simulink model "CMPE243finalprojectdesign0x2DYi0x011Fit_Avar"  (R2023b)
settings: Solver=VariableStepAuto  StartTime=0.0  StopTime=10000  RelTol=1e-3
libraries: simulink_extras x6, embmathops x2, hdlsllib x1
settings Model: PacingRate=5  Creator=berkenulusoy  LastModifiedBy=ASUS TUF

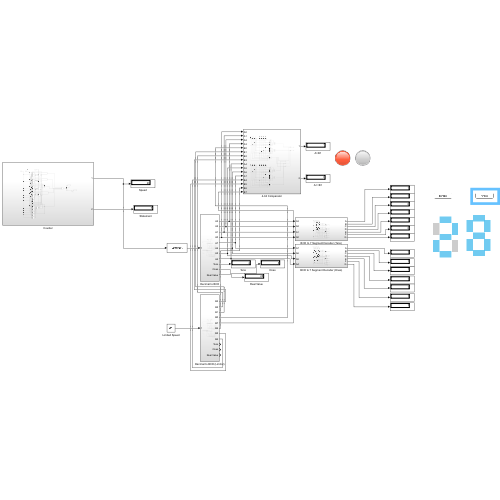
[thumbnail: Simulink's stored preview of the top-level diagram]
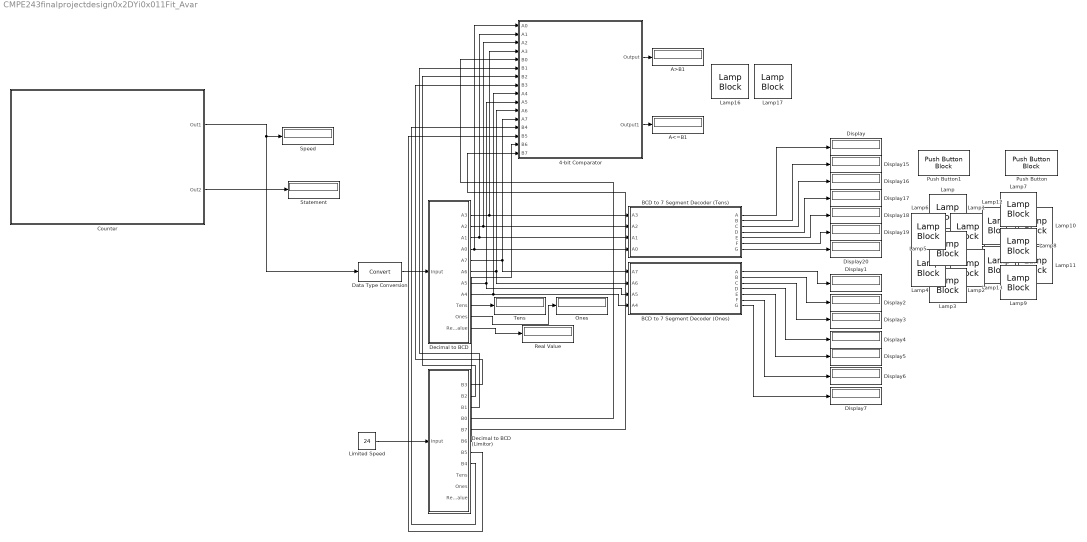
== system CMPE243finalprojectdesign0x2DYi0x011Fit_Avar ==
  4-bit Comparator : Subsystem
  A<=B1 : Display
  A>B1 : Display
  BCD to 7 Segment Decoder (Ones) : Subsystem
  BCD to 7 Segment Decoder (Tens) : Subsystem
  Counter : Subsystem
  Data Type Conversion : DataTypeConversion  SaturateOnIntegerOverflow=off  RndMeth=Floor
  Decimal to BCD : Subsystem
  Decimal to BCD (Limitor) : Subsystem
  Display{,1..7,15..20} (14 alike) : Display
  Lamp{,1..13} (14 alike) : LampBlock  LabelPosition=Hide  Icon=Rectangle
  Lamp16 : LampBlock  LabelPosition=Hide
  Lamp17 : LampBlock  LabelPosition=Hide
  Limited Speed : Constant  Value=24
  Ones : Display
  Push Button : PushButtonBlock  ButtonText=increase  OffValue=0.000000
  Push Button1 : PushButtonBlock  ButtonText=decrease  OffValue=0.000000
  Real Value : Display
  Speed : Display
  Statement : Display
  Tens : Display
  wires:
  Decimal to BCD/9(Tens) -> Tens/1
  Decimal to BCD/10(Ones) -> Ones/1
  Decimal to BCD/11(Real Value) -> Real Value/1
  BCD to 7 Segment Decoder (Ones)/6(F) -> Display6/1
  BCD to 7 Segment Decoder (Tens)/2(B) -> Display15/1
  BCD to 7 Segment Decoder (Ones)/2(B) -> Display2/1
  BCD to 7 Segment Decoder (Ones)/1(A) -> Display1/1
  BCD to 7 Segment Decoder (Tens)/7(G) -> Display20/1
  BCD to 7 Segment Decoder (Ones)/5(E) -> Display5/1
  BCD to 7 Segment Decoder (Ones)/4(D) -> Display4/1
  BCD to 7 Segment Decoder (Ones)/7(G) -> Display7/1
  BCD to 7 Segment Decoder (Tens)/1(A) -> Display/1
  BCD to 7 Segment Decoder (Tens)/5(E) -> Display18/1
  BCD to 7 Segment Decoder (Tens)/3(C) -> Display16/1
  BCD to 7 Segment Decoder (Tens)/4(D) -> Display17/1
  BCD to 7 Segment Decoder (Tens)/6(F) -> Display19/1
  BCD to 7 Segment Decoder (Ones)/3(C) -> Display3/1
  Decimal to BCD/1(A3) -> 4-bit Comparator/4(A3), BCD to 7 Segment Decoder (Tens)/1(A3)
  Decimal to BCD/2(A2) -> 4-bit Comparator/3(A2), BCD to 7 Segment Decoder (Tens)/2(A2)
  Decimal to BCD/4(A0) -> 4-bit Comparator/1(A0), BCD to 7 Segment Decoder (Tens)/4(A0)
  Decimal to BCD/5(A7) -> 4-bit Comparator/12(A7), BCD to 7 Segment Decoder (Ones)/1(A7)
  Decimal to BCD/6(A6) -> 4-bit Comparator/11(A6), BCD to 7 Segment Decoder (Ones)/2(A6)
  Decimal to BCD/7(A5) -> 4-bit Comparator/10(A5), BCD to 7 Segment Decoder (Ones)/3(A5)
  Decimal to BCD/8(A4) -> 4-bit Comparator/9(A4), BCD to 7 Segment Decoder (Ones)/4(A4)
  4-bit Comparator/2(Output1) -> A<=B1/1
  4-bit Comparator/1(Output) -> A>B1/1
  Decimal to BCD/3(A1) -> 4-bit Comparator/2(A1), BCD to 7 Segment Decoder (Tens)/3(A1)
  Data Type Conversion/1 -> Decimal to BCD/1(Input)
  Counter/2(Out2) -> Statement/1
  Counter/1(Out1) -> Data Type Conversion/1, Speed/1
  Decimal to BCD (Limitor)/1(B3) -> 4-bit Comparator/8(B3)
  Decimal to BCD (Limitor)/2(B2) -> 4-bit Comparator/7(B2)
  Decimal to BCD (Limitor)/3(B1) -> 4-bit Comparator/6(B1)
  Decimal to BCD (Limitor)/4(B0) -> 4-bit Comparator/5(B0)
  Decimal to BCD (Limitor)/5(B7) -> 4-bit Comparator/16(B7)
  Decimal to BCD (Limitor)/6(B6) -> 4-bit Comparator/15(B6)
  Decimal to BCD (Limitor)/7(B5) -> 4-bit Comparator/14(B5)
  Decimal to BCD (Limitor)/8(B4) -> 4-bit Comparator/13(B4)
  Limited Speed/1 -> Decimal to BCD (Limitor)/1(Input)

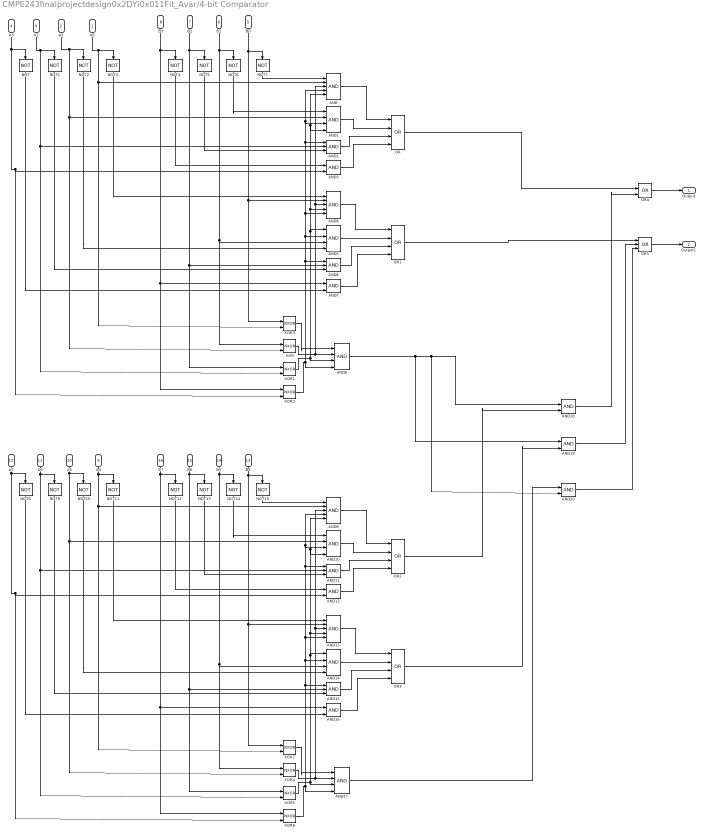
== system CMPE243finalprojectdesign0x2DYi0x011Fit_Avar/4-bit Comparator ==
  A0 : Inport
  A1 : Inport  Port=2
  A2 : Inport  Port=3
  A3 : Inport  Port=4
  B0 : Inport  Port=5
  B1 : Inport  Port=6
  B2 : Inport  Port=7
  B3 : Inport  Port=8
  A4 : Inport  Port=9
  A5 : Inport  Port=10
  A6 : Inport  Port=11
  A7 : Inport  Port=12
  B4 : Inport  Port=13
  B5 : Inport  Port=14
  B6 : Inport  Port=15
  B7 : Inport  Port=16
  AND{,4,9,13} (4 alike) : Logic  Inputs=5  IconShape=distinctive  AllPortsSameDT=off  OutDataTypeStr=boolean
  AND{1,5,8,10,14,17} (6 alike) : Logic  Inputs=4  IconShape=distinctive  AllPortsSameDT=off  OutDataTypeStr=boolean
  AND{2,6,11,15} (4 alike) : Logic  Inputs=3  IconShape=distinctive  AllPortsSameDT=off  OutDataTypeStr=boolean
  AND{3,7,12,16,18..20} (7 alike) : Logic  IconShape=distinctive  AllPortsSameDT=off  OutDataTypeStr=boolean
  NOT{,1..15} (16 alike) : Logic  Operator=NOT  IconShape=distinctive  AllPortsSameDT=off  OutDataTypeStr=boolean
  OR{,1..3} (4 alike) : Logic  Operator=OR  Inputs=4  IconShape=distinctive  AllPortsSameDT=off  OutDataTypeStr=boolean
  OR4 : Logic  Operator=OR  IconShape=distinctive  AllPortsSameDT=off  OutDataTypeStr=boolean
  OR5 : Logic  Operator=OR  Inputs=3  IconShape=distinctive  AllPortsSameDT=off  OutDataTypeStr=boolean
  XOR{,1..7} (8 alike) : Logic  Operator=NXOR  IconShape=distinctive  AllPortsSameDT=off  OutDataTypeStr=boolean
  Output : Outport
  Output1 : Outport  Port=2
  wires:
  NOT12/1 -> AND12/1
  AND12/1 -> OR2/4
  NOT14/1 -> AND10/1
  AND9/1 -> OR2/1
  XOR3/1 -> AND8/1
  OR1/1 -> OR5/1
  AND17/1 -> AND20/1
  AND16/1 -> OR3/4
  AND1/1 -> OR/2
  NOT1/1 -> AND6/3
  NOT11/1 -> AND13/1
  XOR7/1 -> AND17/1
  B1/1 -> NOT6/1, XOR/1, AND5/3
  AND2/1 -> OR/3
  B4/1 -> NOT15/1, XOR7/1, AND13/2
  B7/1 -> NOT12/1, XOR6/1, AND16/1
  NOT4/1 -> AND3/1
  AND4/1 -> OR1/1
  OR/1 -> OR4/1
  NOT9/1 -> AND15/3
  NOT5/1 -> AND2/3
  AND14/1 -> OR3/2
  OR3/1 -> AND19/2
  XOR/1 -> AND8/2, AND4/3, AND/3
  NOT7/1 -> AND/1
  A6/1 -> NOT9/1, XOR5/2, AND11/2
  NOT3/1 -> AND4/1
  A7/1 -> NOT8/1, XOR6/2, AND12/2
  OR5/1 -> Output1/1
  NOT8/1 -> AND16/2
  A2/1 -> NOT1/1, XOR1/2, AND2/2
  AND5/1 -> OR1/2
  XOR5/1 -> AND14/1, AND13/4, AND10/4, AND9/5, AND17/3
  NOT13/1 -> AND11/3
  AND6/1 -> OR1/3
  AND3/1 -> OR/4
  B3/1 -> NOT4/1, XOR2/1, AND7/1
  AND15/1 -> OR3/3
  B2/1 -> NOT5/1, XOR1/1, AND6/2
  AND8/1 -> AND19/1, AND20/2, AND18/1
  NOT/1 -> AND7/2
  AND10/1 -> OR2/2
  A4/1 -> NOT11/1, XOR7/2, AND9/2
  NOT15/1 -> AND9/1
  AND7/1 -> OR1/4
  A5/1 -> NOT10/1, XOR4/2, AND10/2
  XOR6/1 -> AND17/4, AND15/1, AND14/2, AND13/5, AND11/1, AND10/3, AND9/4
  B0/1 -> NOT7/1, XOR3/1, AND4/2
  NOT6/1 -> AND1/1
  AND/1 -> OR/1
  A0/1 -> NOT3/1, XOR3/2, AND/2
  A3/1 -> NOT/1, XOR2/2, AND3/2
  NOT10/1 -> AND14/4
  OR2/1 -> AND18/2
  AND19/1 -> OR5/2
  B5/1 -> NOT14/1, XOR4/1, AND14/3
  B6/1 -> NOT13/1, XOR5/1, AND15/2
  AND13/1 -> OR3/1
  XOR4/1 -> AND17/2, AND13/3, AND9/3
  XOR1/1 -> AND5/1, AND4/4, AND1/4, AND/5, AND8/3
  XOR2/1 -> AND8/4, AND6/1, AND5/2, AND4/5, AND2/1, AND1/3, AND/4
  OR4/1 -> Output/1
  AND11/1 -> OR2/3
  A1/1 -> NOT2/1, XOR/2, AND1/2
  AND18/1 -> OR4/2
  NOT2/1 -> AND5/4
  AND20/1 -> OR5/3

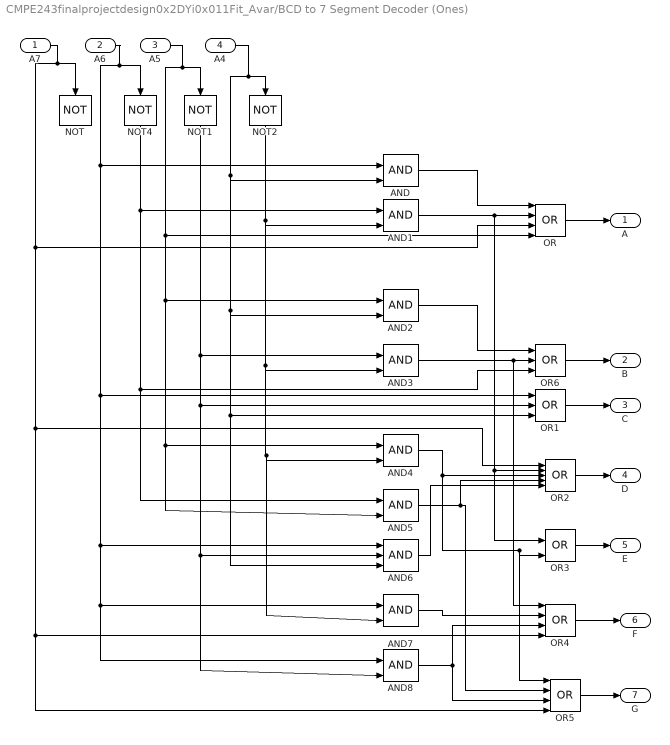
== system CMPE243finalprojectdesign0x2DYi0x011Fit_Avar/BCD to 7 Segment Decoder (Ones) ==
  A7 : Inport
  A6 : Inport  Port=2
  A5 : Inport  Port=3
  A4 : Inport  Port=4
  AND{,1..5,7..8} (8 alike) : Logic  IconShape=distinctive  AllPortsSameDT=off  OutDataTypeStr=boolean
  AND6 : Logic  Inputs=3  IconShape=distinctive  AllPortsSameDT=off  OutDataTypeStr=boolean
  NOT{,1..2,4} (4 alike) : Logic  Operator=NOT  IconShape=distinctive  AllPortsSameDT=off  OutDataTypeStr=boolean
  OR : Logic  Operator=OR  Inputs=4  IconShape=distinctive  AllPortsSameDT=off  OutDataTypeStr=boolean
  OR1 : Logic  Operator=OR  Inputs=3  IconShape=distinctive  AllPortsSameDT=off  OutDataTypeStr=boolean
  OR2 : Logic  Operator=OR  Inputs=5  IconShape=distinctive  AllPortsSameDT=off  OutDataTypeStr=boolean
  OR3 : Logic  Operator=OR  IconShape=distinctive  AllPortsSameDT=off  OutDataTypeStr=boolean
  OR4 : Logic  Operator=OR  Inputs=4  IconShape=distinctive  AllPortsSameDT=off  OutDataTypeStr=boolean
  OR5 : Logic  Operator=OR  Inputs=4  IconShape=distinctive  AllPortsSameDT=off  OutDataTypeStr=boolean
  OR6 : Logic  Operator=OR  Inputs=3  IconShape=distinctive  AllPortsSameDT=off  OutDataTypeStr=boolean
  A : Outport
  B : Outport  Port=2
  C : Outport  Port=3
  D : Outport  Port=4
  E : Outport  Port=5
  F : Outport  Port=6
  G : Outport  Port=7
  wires:
  OR5/1 -> G/1
  A7/1 -> NOT/1, OR/3, OR4/4, OR5/4, OR2/1
  AND8/1 -> OR4/3, OR5/3
  AND3/1 -> OR4/1, OR6/2
  NOT4/1 -> AND1/1, OR6/3, AND5/1
  AND1/1 -> OR2/2, OR3/1, OR/2
  AND5/1 -> OR2/4, OR5/2
  AND/1 -> OR/1
  AND7/1 -> OR4/2
  OR4/1 -> F/1
  OR6/1 -> B/1
  OR3/1 -> E/1
  NOT2/1 -> AND1/2, AND3/2, AND7/2, AND4/2
  AND2/1 -> OR6/1
  AND6/1 -> OR2/5
  A5/1 -> NOT1/1, OR/4, AND2/1, AND4/1, AND5/2
  OR2/1 -> D/1
  NOT1/1 -> AND3/1, OR1/2, AND6/2, AND8/2
  OR1/1 -> C/1
  A4/1 -> NOT2/1, AND/2, AND2/2, OR1/3, AND6/3
  A6/1 -> NOT4/1, AND/1, OR1/1, AND6/1, AND7/1, AND8/1
  AND4/1 -> OR2/3, OR5/1, OR3/2
  OR/1 -> A/1

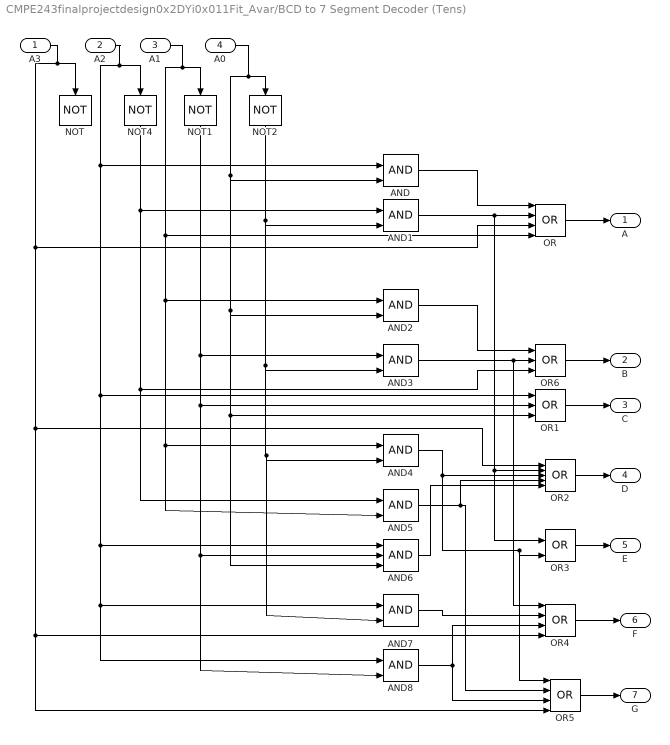
== system CMPE243finalprojectdesign0x2DYi0x011Fit_Avar/BCD to 7 Segment Decoder (Tens) ==
  A3 : Inport
  A2 : Inport  Port=2
  A1 : Inport  Port=3
  A0 : Inport  Port=4
  AND{,1..5,7..8} (8 alike) : Logic  IconShape=distinctive  AllPortsSameDT=off  OutDataTypeStr=boolean
  AND6 : Logic  Inputs=3  IconShape=distinctive  AllPortsSameDT=off  OutDataTypeStr=boolean
  NOT{,1..2,4} (4 alike) : Logic  Operator=NOT  IconShape=distinctive  AllPortsSameDT=off  OutDataTypeStr=boolean
  OR : Logic  Operator=OR  Inputs=4  IconShape=distinctive  AllPortsSameDT=off  OutDataTypeStr=boolean
  OR1 : Logic  Operator=OR  Inputs=3  IconShape=distinctive  AllPortsSameDT=off  OutDataTypeStr=boolean
  OR2 : Logic  Operator=OR  Inputs=5  IconShape=distinctive  AllPortsSameDT=off  OutDataTypeStr=boolean
  OR3 : Logic  Operator=OR  IconShape=distinctive  AllPortsSameDT=off  OutDataTypeStr=boolean
  OR4 : Logic  Operator=OR  Inputs=4  IconShape=distinctive  AllPortsSameDT=off  OutDataTypeStr=boolean
  OR5 : Logic  Operator=OR  Inputs=4  IconShape=distinctive  AllPortsSameDT=off  OutDataTypeStr=boolean
  OR6 : Logic  Operator=OR  Inputs=3  IconShape=distinctive  AllPortsSameDT=off  OutDataTypeStr=boolean
  A : Outport
  B : Outport  Port=2
  C : Outport  Port=3
  D : Outport  Port=4
  E : Outport  Port=5
  F : Outport  Port=6
  G : Outport  Port=7
  wires:
  OR5/1 -> G/1
  A3/1 -> NOT/1, OR/3, OR4/4, OR5/4, OR2/1
  AND8/1 -> OR4/3, OR5/3
  AND3/1 -> OR4/1, OR6/2
  NOT4/1 -> AND1/1, OR6/3, AND5/1
  AND1/1 -> OR2/2, OR3/1, OR/2
  AND5/1 -> OR2/4, OR5/2
  AND/1 -> OR/1
  AND7/1 -> OR4/2
  OR4/1 -> F/1
  OR6/1 -> B/1
  OR3/1 -> E/1
  NOT2/1 -> AND1/2, AND3/2, AND7/2, AND4/2
  AND2/1 -> OR6/1
  AND6/1 -> OR2/5
  A1/1 -> NOT1/1, OR/4, AND2/1, AND4/1, AND5/2
  OR2/1 -> D/1
  NOT1/1 -> AND3/1, OR1/2, AND6/2, AND8/2
  OR1/1 -> C/1
  A0/1 -> NOT2/1, AND/2, AND2/2, OR1/3, AND6/3
  A2/1 -> NOT4/1, AND/1, OR1/1, AND6/1, AND7/1, AND8/1
  AND4/1 -> OR2/3, OR5/1, OR3/2
  OR/1 -> A/1

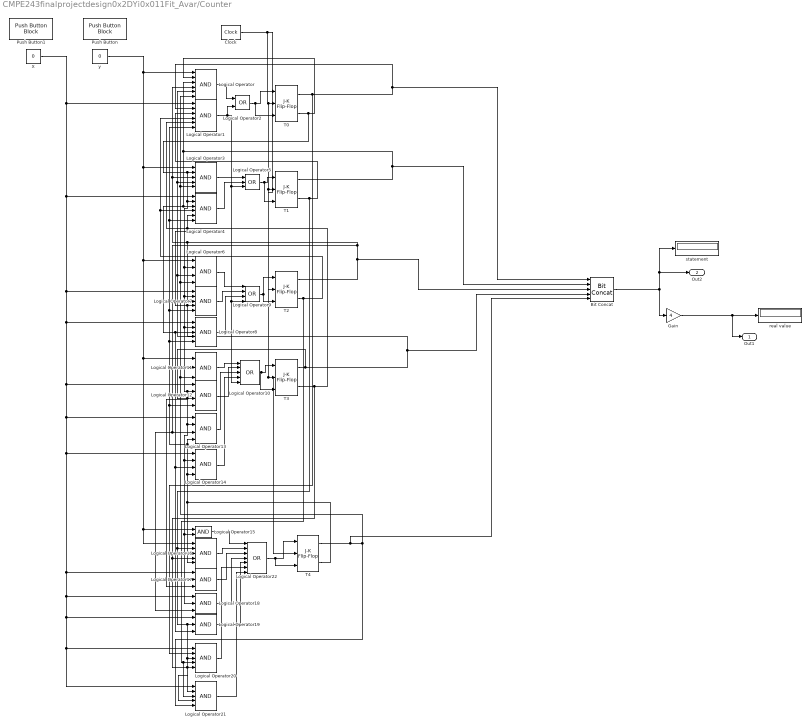
== system CMPE243finalprojectdesign0x2DYi0x011Fit_Avar/Counter ==
  Bit Concat : hdlsllib/Logic and Bit Operations/Bit Concat  numInputs=5
  Clock : simulink_extras/Flip Flops/Clock  period=1
  Gain : Gain  Gain=4
  Logical Operator : Logic  Inputs=6  AllPortsSameDT=off  OutDataTypeStr=boolean
  Logical Operator1 : Logic  Inputs=6  AllPortsSameDT=off  OutDataTypeStr=boolean
  Logical Operator10 : Logic  Operator=OR  Inputs=5  AllPortsSameDT=off  OutDataTypeStr=boolean
  Logical Operator{11,17..19} (4 alike) : Logic  Inputs=3  AllPortsSameDT=off  OutDataTypeStr=boolean
  Logical Operator{6,12..14} (4 alike) : Logic  Inputs=4  AllPortsSameDT=off  OutDataTypeStr=boolean
  Logical Operator15 : Logic  AllPortsSameDT=off  OutDataTypeStr=boolean
  Logical Operator{3,7..8,16,20..21} (6 alike) : Logic  Inputs=5  AllPortsSameDT=off  OutDataTypeStr=boolean
  Logical Operator2 : Logic  Operator=OR  AllPortsSameDT=off  OutDataTypeStr=boolean
  Logical Operator22 : Logic  Operator=OR  Inputs=7  AllPortsSameDT=off  OutDataTypeStr=boolean
  Logical Operator4 : Logic  Inputs=6  AllPortsSameDT=off  OutDataTypeStr=boolean
  Logical Operator5 : Logic  Operator=OR  Inputs=3  AllPortsSameDT=off  OutDataTypeStr=boolean
  Logical Operator9 : Logic  Operator=OR  Inputs=4  AllPortsSameDT=off  OutDataTypeStr=boolean
  Push Button : PushButtonBlock  ButtonText=increase  OffValue=0.000000
  Push Button1 : PushButtonBlock  ButtonText=decrease  OffValue=0.000000
  T{0..4} (5 alike) : simulink_extras/Flip Flops/J-K Flip-Flop  initial_condition=0
  X : Constant  Value=0
  real value : Display
  statement : Display
  y : Constant  Value=0
  Out1 : Outport
  Out2 : Outport  Port=2
  wires:
  X/1 -> Logical Operator1/1, Logical Operator4/1, Logical Operator7/1, Logical Operator8/1, Logical Operator12/1, Logical Operator13/1, Logical Operator14/1, Logical Operator17/1, Logical Operator19/1, Logical Operator21/1, Logical Operator20/1, Logical Operator18/1
  y/1 -> Logical Operator/1, Logical Operator3/1, Logical Operator6/1, Logical Operator11/1, Logical Operator15/1, Logical Operator16/1
  Logical Operator/1 -> Logical Operator2/1
  Logical Operator2/1 -> T0/3, T0/1
  T0/2 -> Logical Operator4/2, Logical Operator18/2, Logical Operator17/2, Logical Operator15/2, Logical Operator14/2, Logical Operator13/2, Logical Operator12/2, Logical Operator11/2, Logical Operator8/2, Logical Operator7/2, Logical Operator6/2, Logical Operator3/2, Logical Operator/2
  T1/2 -> Logical Operator16/2, Logical Operator21/2, Logical Operator20/3, Logical Operator19/2, Logical Operator1/3
  T2/2 -> Logical Operator16/3, Logical Operator20/4, Logical Operator21/3, Logical Operator4/4, Logical Operator1/4
  T3/2 -> Logical Operator16/4, Logical Operator21/4, Logical Operator20/5, Logical Operator8/4, Logical Operator7/4, Logical Operator1/5, Logical Operator4/5
  T4/2 -> Logical Operator16/5, Logical Operator12/4, Logical Operator8/5, Logical Operator7/5, Logical Operator4/6, Logical Operator1/6, Logical Operator13/4, Logical Operator14/4
  Logical Operator1/1 -> Logical Operator2/2, Logical Operator5/3, Logical Operator10/5, Logical Operator9/4
  Logical Operator3/1 -> Logical Operator5/1
  Logical Operator4/1 -> Logical Operator5/2
  Logical Operator5/1 -> T1/3, T1/1
  Logical Operator6/1 -> Logical Operator9/1
  Logical Operator7/1 -> Logical Operator9/2
  Logical Operator8/1 -> Logical Operator9/3
  Logical Operator9/1 -> T2/1, T2/3
  Logical Operator10/1 -> T3/3, T3/1
  Logical Operator11/1 -> Logical Operator10/1
  Logical Operator12/1 -> Logical Operator10/2
  Logical Operator13/1 -> Logical Operator10/3
  Logical Operator14/1 -> Logical Operator10/4
  Logical Operator15/1 -> Logical Operator22/1
  Logical Operator16/1 -> Logical Operator22/2
  Logical Operator17/1 -> Logical Operator22/3
  Logical Operator18/1 -> Logical Operator22/4
  Logical Operator19/1 -> Logical Operator22/5
  Logical Operator20/1 -> Logical Operator22/6
  Logical Operator21/1 -> Logical Operator22/7
  Logical Operator22/1 -> T4/1, T4/3
  Clock/1 -> T2/2, T1/2, T4/2, T3/2, T0/2
  T0/1 -> Logical Operator20/2, Bit Concat/1, Logical Operator1/2
  T1/1 -> Bit Concat/2, Logical Operator8/3, Logical Operator14/3, Logical Operator19/3, Logical Operator4/3, Logical Operator/3
  T2/1 -> Bit Concat/3, Logical Operator13/3, Logical Operator18/3, Logical Operator7/3, Logical Operator3/3, Logical Operator/4
  T3/1 -> Logical Operator17/3, Logical Operator12/3, Bit Concat/4, Logical Operator6/3, Logical Operator3/4, Logical Operator/5
  T4/1 -> Bit Concat/5, Logical Operator21/5, Logical Operator11/3, Logical Operator6/4, Logical Operator3/5, Logical Operator/6
  Bit Concat/1 -> statement/1, Out2/1, Gain/1
  Gain/1 -> Out1/1, real value/1

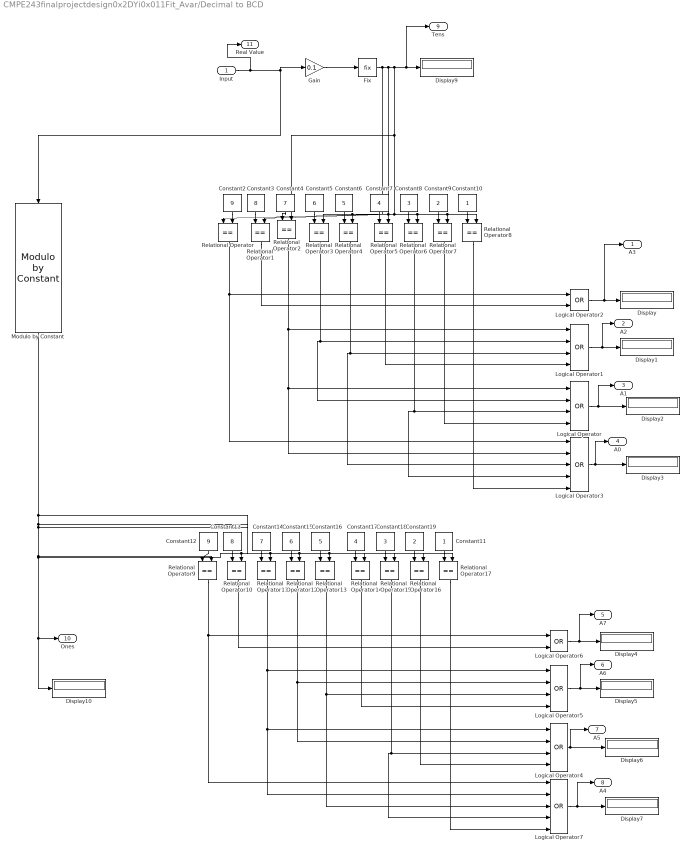
== system CMPE243finalprojectdesign0x2DYi0x011Fit_Avar/Decimal to BCD ==
  Input : Inport
  Constant10 : Constant
  Constant11 : Constant
  Constant12 : Constant  Value=9
  Constant13 : Constant  Value=8
  Constant14 : Constant  Value=7
  Constant15 : Constant  Value=6
  Constant16 : Constant  Value=5
  Constant17 : Constant  Value=4
  Constant18 : Constant  Value=3
  Constant19 : Constant  Value=2
  Constant2 : Constant  Value=9
  Constant3 : Constant  Value=8
  Constant4 : Constant  Value=7
  Constant5 : Constant  Value=6
  Constant6 : Constant  Value=5
  Constant7 : Constant  Value=4
  Constant8 : Constant  Value=3
  Constant9 : Constant  Value=2
  Display{,1..7,9..10} (10 alike) : Display
  Fix : Rounding  Operator=fix
  Gain : Gain  Gain=0.1
  Logical Operator{,1,4..5} (4 alike) : Logic  Operator=OR  Inputs=4  AllPortsSameDT=off  OutDataTypeStr=boolean
  Logical Operator2 : Logic  Operator=OR  AllPortsSameDT=off  OutDataTypeStr=boolean
  Logical Operator3 : Logic  Operator=OR  Inputs=5  AllPortsSameDT=off  OutDataTypeStr=boolean
  Logical Operator6 : Logic  Operator=OR  AllPortsSameDT=off  OutDataTypeStr=boolean
  Logical Operator7 : Logic  Operator=OR  Inputs=5  AllPortsSameDT=off  OutDataTypeStr=boolean
  Modulo by Constant : embmathops/Modulo by Constant  Denominator=10  SimulateUsing=Code generation
      settings: LibrarySourceBlock=embeddedMathLib/Modulo by Constant
  Relational Operator{,1..17} (18 alike) : RelationalOperator  Operator===  OutDataTypeStr=boolean  RndMeth=Simplest  InputSameDT=off
  A3 : Outport
  A2 : Outport  Port=2
  A1 : Outport  Port=3
  A0 : Outport  Port=4
  A7 : Outport  Port=5
  A6 : Outport  Port=6
  A5 : Outport  Port=7
  A4 : Outport  Port=8
  Tens : Outport  Port=9
  Ones : Outport  Port=10
  Real Value : Outport  Port=11
  wires:
  Constant11/1 -> Relational Operator17/1
  Relational Operator10/1 -> Logical Operator6/2
  Relational Operator7/1 -> Logical Operator/4
  Fix/1 -> Relational Operator8/2, Relational Operator7/2, Relational Operator6/2, Relational Operator5/2, Relational Operator4/2, Relational Operator3/2, Relational Operator2/2, Tens/1, Display9/1, Relational Operator1/2, Relational Operator/1
  Relational Operator13/1 -> Logical Operator5/3, Logical Operator7/3
  Relational Operator/1 -> Logical Operator2/1, Logical Operator3/1
  Constant18/1 -> Relational Operator15/1
  Constant7/1 -> Relational Operator5/1
  Logical Operator2/1 -> A3/1, Display/1
  Logical Operator4/1 -> A5/1, Display6/1
  Constant10/1 -> Relational Operator8/1
  Relational Operator1/1 -> Logical Operator2/2
  Input/1 -> Real Value/1, Gain/1, Modulo by Constant/1
  Logical Operator1/1 -> A2/1, Display1/1
  Relational Operator6/1 -> Logical Operator3/4, Logical Operator/3
  Constant17/1 -> Relational Operator14/1
  Relational Operator12/1 -> Logical Operator5/2, Logical Operator4/2
  Constant8/1 -> Relational Operator6/1
  Constant6/1 -> Relational Operator4/1
  Constant15/1 -> Relational Operator12/1
  Relational Operator14/1 -> Logical Operator5/4
  Logical Operator5/1 -> A6/1, Display5/1
  Relational Operator15/1 -> Logical Operator7/4, Logical Operator4/3
  Relational Operator2/1 -> Logical Operator1/1, Logical Operator/1, Logical Operator3/2
  Constant5/1 -> Relational Operator3/1
  Constant19/1 -> Relational Operator16/1
  Constant13/1 -> Relational Operator10/1
  Logical Operator/1 -> A1/1, Display2/1
  Relational Operator5/1 -> Logical Operator1/4
  Constant9/1 -> Relational Operator7/1
  Relational Operator11/1 -> Logical Operator5/1, Logical Operator4/1, Logical Operator7/2
  Constant16/1 -> Relational Operator13/1
  Logical Operator7/1 -> A4/1, Display7/1
  Gain/1 -> Fix/1
  Relational Operator17/1 -> Logical Operator7/5
  Logical Operator6/1 -> A7/1, Display4/1
  Relational Operator8/1 -> Logical Operator3/5
  Relational Operator3/1 -> Logical Operator/2, Logical Operator1/2
  Logical Operator3/1 -> A0/1, Display3/1
  Relational Operator4/1 -> Logical Operator3/3, Logical Operator1/3
  Constant12/1 -> Relational Operator9/1
  Constant3/1 -> Relational Operator1/1
  Constant4/1 -> Relational Operator2/1
  Constant14/1 -> Relational Operator11/1
  Modulo by Constant/1 -> Relational Operator16/2, Relational Operator15/2, Relational Operator14/2, Relational Operator17/2, Relational Operator13/2, Relational Operator12/2, Relational Operator11/2, Relational Operator10/2, Ones/1, Display10/1, Relational Operator9/2
  Relational Operator16/1 -> Logical Operator4/4
  Constant2/1 -> Relational Operator/2
  Relational Operator9/1 -> Logical Operator6/1, Logical Operator7/1

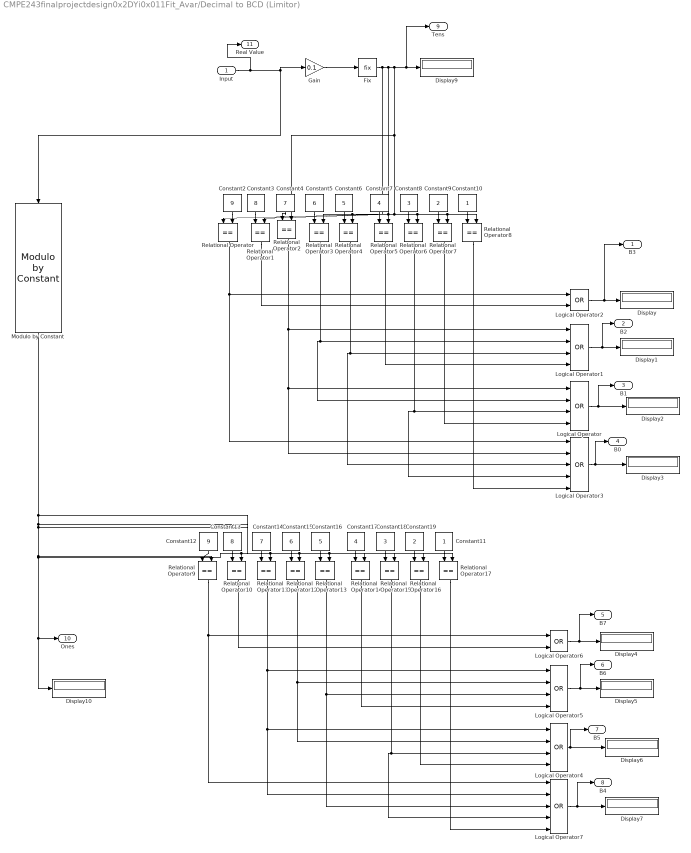
== system CMPE243finalprojectdesign0x2DYi0x011Fit_Avar/Decimal to BCD (Limitor) ==
  Input : Inport
  Constant10 : Constant
  Constant11 : Constant
  Constant12 : Constant  Value=9
  Constant13 : Constant  Value=8
  Constant14 : Constant  Value=7
  Constant15 : Constant  Value=6
  Constant16 : Constant  Value=5
  Constant17 : Constant  Value=4
  Constant18 : Constant  Value=3
  Constant19 : Constant  Value=2
  Constant2 : Constant  Value=9
  Constant3 : Constant  Value=8
  Constant4 : Constant  Value=7
  Constant5 : Constant  Value=6
  Constant6 : Constant  Value=5
  Constant7 : Constant  Value=4
  Constant8 : Constant  Value=3
  Constant9 : Constant  Value=2
  Display{,1..7,9..10} (10 alike) : Display
  Fix : Rounding  Operator=fix
  Gain : Gain  Gain=0.1
  Logical Operator{,1,4..5} (4 alike) : Logic  Operator=OR  Inputs=4  AllPortsSameDT=off  OutDataTypeStr=boolean
  Logical Operator2 : Logic  Operator=OR  AllPortsSameDT=off  OutDataTypeStr=boolean
  Logical Operator3 : Logic  Operator=OR  Inputs=5  AllPortsSameDT=off  OutDataTypeStr=boolean
  Logical Operator6 : Logic  Operator=OR  AllPortsSameDT=off  OutDataTypeStr=boolean
  Logical Operator7 : Logic  Operator=OR  Inputs=5  AllPortsSameDT=off  OutDataTypeStr=boolean
  Modulo by Constant : embmathops/Modulo by Constant  Denominator=10  SimulateUsing=Code generation
      settings: LibrarySourceBlock=embeddedMathLib/Modulo by Constant
  Relational Operator{,1..17} (18 alike) : RelationalOperator  Operator===  OutDataTypeStr=boolean  RndMeth=Simplest  InputSameDT=off
  B3 : Outport
  B2 : Outport  Port=2
  B1 : Outport  Port=3
  B0 : Outport  Port=4
  B7 : Outport  Port=5
  B6 : Outport  Port=6
  B5 : Outport  Port=7
  B4 : Outport  Port=8
  Tens : Outport  Port=9
  Ones : Outport  Port=10
  Real Value : Outport  Port=11
  wires:
  Constant11/1 -> Relational Operator17/1
  Relational Operator10/1 -> Logical Operator6/2
  Relational Operator7/1 -> Logical Operator/4
  Fix/1 -> Relational Operator8/2, Relational Operator7/2, Relational Operator6/2, Relational Operator5/2, Relational Operator4/2, Relational Operator3/2, Relational Operator2/2, Tens/1, Display9/1, Relational Operator1/2, Relational Operator/1
  Relational Operator13/1 -> Logical Operator5/3, Logical Operator7/3
  Relational Operator/1 -> Logical Operator2/1, Logical Operator3/1
  Constant18/1 -> Relational Operator15/1
  Constant7/1 -> Relational Operator5/1
  Logical Operator2/1 -> B3/1, Display/1
  Logical Operator4/1 -> B5/1, Display6/1
  Constant10/1 -> Relational Operator8/1
  Relational Operator1/1 -> Logical Operator2/2
  Input/1 -> Real Value/1, Gain/1, Modulo by Constant/1
  Logical Operator1/1 -> B2/1, Display1/1
  Relational Operator6/1 -> Logical Operator3/4, Logical Operator/3
  Constant17/1 -> Relational Operator14/1
  Relational Operator12/1 -> Logical Operator5/2, Logical Operator4/2
  Constant8/1 -> Relational Operator6/1
  Constant6/1 -> Relational Operator4/1
  Constant15/1 -> Relational Operator12/1
  Relational Operator14/1 -> Logical Operator5/4
  Logical Operator5/1 -> B6/1, Display5/1
  Relational Operator15/1 -> Logical Operator7/4, Logical Operator4/3
  Relational Operator2/1 -> Logical Operator1/1, Logical Operator/1, Logical Operator3/2
  Constant5/1 -> Relational Operator3/1
  Constant19/1 -> Relational Operator16/1
  Constant13/1 -> Relational Operator10/1
  Logical Operator/1 -> B1/1, Display2/1
  Relational Operator5/1 -> Logical Operator1/4
  Constant9/1 -> Relational Operator7/1
  Relational Operator11/1 -> Logical Operator5/1, Logical Operator4/1, Logical Operator7/2
  Constant16/1 -> Relational Operator13/1
  Logical Operator7/1 -> B4/1, Display7/1
  Gain/1 -> Fix/1
  Relational Operator17/1 -> Logical Operator7/5
  Logical Operator6/1 -> B7/1, Display4/1
  Relational Operator8/1 -> Logical Operator3/5
  Relational Operator3/1 -> Logical Operator/2, Logical Operator1/2
  Logical Operator3/1 -> B0/1, Display3/1
  Relational Operator4/1 -> Logical Operator3/3, Logical Operator1/3
  Constant12/1 -> Relational Operator9/1
  Constant3/1 -> Relational Operator1/1
  Constant4/1 -> Relational Operator2/1
  Constant14/1 -> Relational Operator11/1
  Modulo by Constant/1 -> Relational Operator16/2, Relational Operator15/2, Relational Operator14/2, Relational Operator17/2, Relational Operator13/2, Relational Operator12/2, Relational Operator11/2, Relational Operator10/2, Ones/1, Display10/1, Relational Operator9/2
  Relational Operator16/1 -> Logical Operator4/4
  Constant2/1 -> Relational Operator/2
  Relational Operator9/1 -> Logical Operator6/1, Logical Operator7/1
